simulink model "Rotation_test"  (Simulink 7.4)
settings: Solver=ode45  StartTime=0.0  StopTime=10.0  RelTol=1e-3
settings Model: Creator=roczit00  LastModifiedBy=roczit00

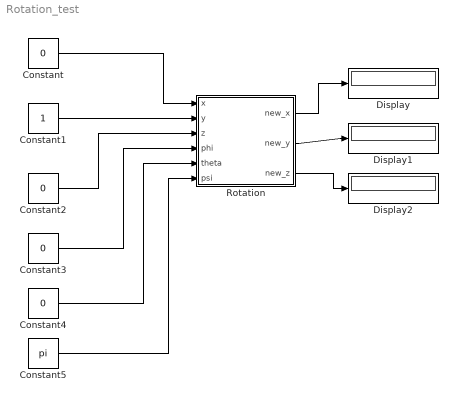
== system Rotation_test ==
  Constant{,2..4} (4 alike) : Constant  Value=0  OutDataType=fixdt(1, 16)  OutScaling=2^0
  Constant1 : Constant  OutDataType=fixdt(1, 16)  OutScaling=2^0
  Constant5 : Constant  Value=pi  OutDataType=fixdt(1, 16)  OutScaling=2^0
  Display : Display
  Display1 : Display
  Display2 : Display
  Rotation : Subsystem
  wires:
  Constant/1 -> Rotation/1(x)
  Constant1/1 -> Rotation/2(y)
  Constant2/1 -> Rotation/3(z)
  Rotation/1(new_x) -> Display/1
  Rotation/2(new_y) -> Display1/1
  Rotation/3(new_z) -> Display2/1
  Constant3/1 -> Rotation/4(phi)
  Constant4/1 -> Rotation/5(theta)
  Constant5/1 -> Rotation/6(psi)

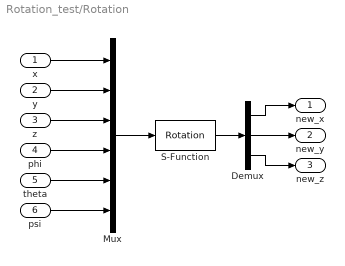
== system Rotation_test/Rotation ==
  x : Inport  OutDataType=fixdt(1, 16)  OutScaling=2^0
  y : Inport  Port=2  OutDataType=fixdt(1, 16)  OutScaling=2^0
  z : Inport  Port=3  OutDataType=fixdt(1, 16)  OutScaling=2^0
  phi : Inport  Port=4  OutDataType=fixdt(1, 16)  OutScaling=2^0
  theta : Inport  Port=5  OutDataType=fixdt(1, 16)  OutScaling=2^0
  psi : Inport  Port=6  OutDataType=fixdt(1, 16)  OutScaling=2^0
  Demux : Demux  Outputs=3
  Mux : Mux  Inputs=6
  S-Function : S-Function  FunctionName=Rotation  EnableBusSupport=off
  new_x : Outport  OutDataType=fixdt(1, 16)  OutScaling=2^0
  new_y : Outport  Port=2  OutDataType=fixdt(1, 16)  OutScaling=2^0
  new_z : Outport  Port=3  OutDataType=fixdt(1, 16)  OutScaling=2^0
  wires:
  x/1 -> Mux/1
  y/1 -> Mux/2
  z/1 -> Mux/3
  Mux/1 -> S-Function/1
  S-Function/1 -> Demux/1
  Demux/2 -> new_y/1
  Demux/1 -> new_x/1
  Demux/3 -> new_z/1
  phi/1 -> Mux/4
  theta/1 -> Mux/5
  psi/1 -> Mux/6
